simulink model "chap2_6sim"  (R2015a)
settings: Solver=ode45  SolverMode=SingleTasking  StartTime=0.0  StopTime=RunTime  RelTol=1e-3
settings Model: Creator=Masoud  LastModifiedBy=MSD
settings OptimizationCC: BlockReduction=off  BooleanDataType=off
settings DebuggingCC: AlgebraicLoopMsg=none  SaveWithParameterizedLinksMsg=none  UnderspecifiedInitializationDetection=Classic  MergeDetectMultiDrivingBlocksExec=none  SignalResolutionControl=TryResolveAllWithWarning  InheritedTsInSrcMsg=none  DiscreteInheritContinuousMsg=none
settings HardwareCC: TargetUnknown=on

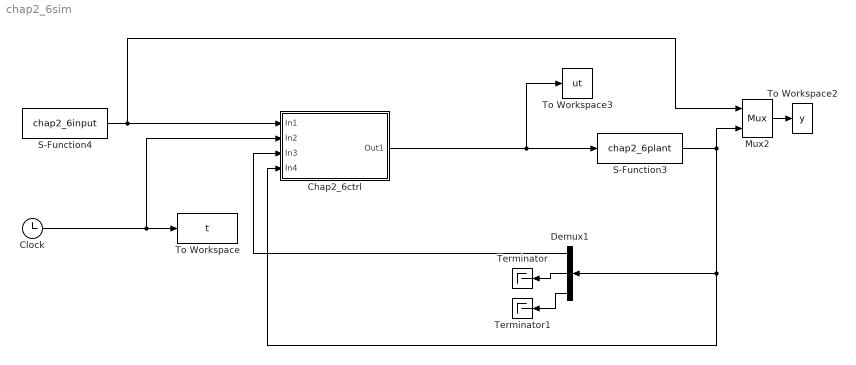
== system chap2_6sim ==
  Chap2_6ctrl : Subsystem
  Clock : Clock
  Demux1 : Demux  Outputs=3
  Mux2 : Mux  Inputs=2
  S-Function3 : S-Function  FunctionName=chap2_6plant  SFunctionModules='chap2_6plant'
  S-Function4 : S-Function  FunctionName=chap2_6input  SFunctionModules='chap2_6input'
  Terminator : Terminator
  Terminator1 : Terminator
  To Workspace : ToWorkspace  VariableName=t  SampleTime=-1
  To Workspace2 : ToWorkspace  VariableName=y  SampleTime=-1
  To Workspace3 : ToWorkspace  VariableName=ut  SampleTime=-1
  wires:
  Mux2/1 -> To Workspace2/1
  Demux1/2 -> Terminator/1
  Demux1/3 -> Terminator1/1
  Chap2_6ctrl/1(Out1) -> S-Function3/1, To Workspace3/1
  S-Function4/1 -> Mux2/1, Chap2_6ctrl/1(In1)
  S-Function3/1 -> Mux2/2, Chap2_6ctrl/4(In4), Demux1/1
  Demux1/1 -> Chap2_6ctrl/3(In3)
  Clock/1 -> Chap2_6ctrl/2(In2), To Workspace/1

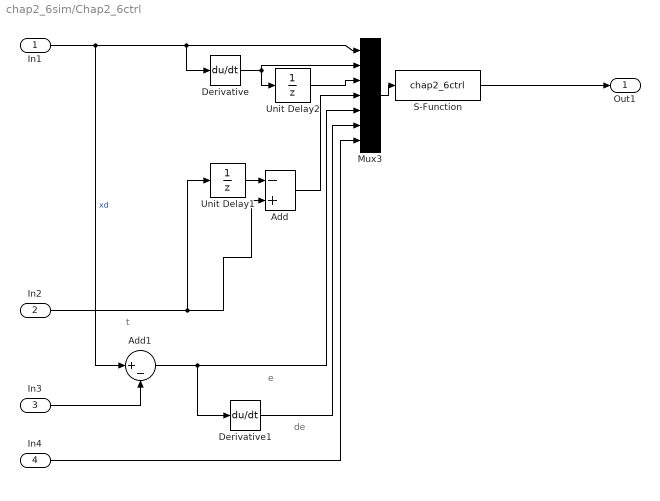
== system chap2_6sim/Chap2_6ctrl ==
  note: t
  note: de
  note: e
  In1 : Inport
  In2 : Inport  Port=2
  In3 : Inport  Port=3
  In4 : Inport  Port=4
  Add : Sum  Inputs=-+
  Add1 : Sum  Inputs=|+-
  Derivative : Derivative
  Derivative1 : Derivative
  Mux3 : Mux  Inputs=7
  S-Function : S-Function  FunctionName=chap2_6ctrl  SFunctionModules='chap2_6ctrl'
  Unit Delay1 : UnitDelay  SampleTime=-1
  Unit Delay2 : UnitDelay  SampleTime=-1
  Out1 : Outport
  wires:
  S-Function/1 -> Out1/1
  In2/1 -> Add/2, Unit Delay1/1
  In4/1 -> Mux3/7
  Unit Delay2/1 -> Mux3/3
  Derivative/1 -> Mux3/2, Unit Delay2/1
  Mux3/1 -> S-Function/1
  Add/1 -> Mux3/4
  In1/1 -> Add1/1, Derivative/1, Mux3/1  "xd"
  Unit Delay1/1 -> Add/1
  Derivative1/1 -> Mux3/6
  In3/1 -> Add1/2
  Add1/1 -> Derivative1/1, Mux3/5
